simulink model "trocador_PS_GPC_sim"  (R2020a)
settings: Solver=VariableStepAuto  StartTime=0.0  StopTime=tsim  MaxStep=0.01  RelTol=1e-3
values from neighbouring files (symbols this model uses):
  amppert = 0.3    [trocador_PS_GPC.m]
  amppert2 = -0.1    [trocador_PS_GPC.m]
  ampref = 0.5    [trocador_PS_GPC.m]
  F = Ftemp    [trocador_PS_GPC.m]
  H = cell2mat(H)    [trocador_PS_GPC.m]
  Kgpc1 = [Kgpc1; Kgpc(sum(Nu(1:i-1))+1,:)]    [trocador_PS_GPC.m]
  tpert = 15    [trocador_PS_GPC.m]
  tpert2 = 25    [trocador_PS_GPC.m]
  tref = 4    [trocador_PS_GPC.m]
  Ts = 0.15    [trocador_PS_GPC.m]
  zr = blkdiag(zr,ones(N(i),1))    [trocador_PS_GPC.m]
libraries: cstblocks x8
settings Model: Creator=treezao  LastModifiedBy=treezao

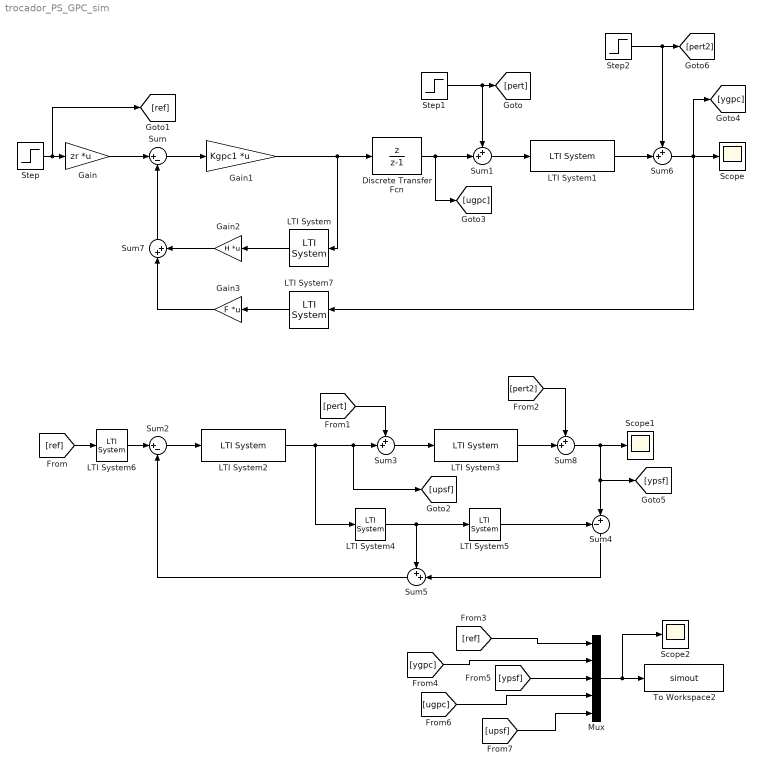
== system trocador_PS_GPC_sim ==
  Discrete Transfer Fcn : DiscreteTransferFcn  Numerator=[1 0]  Denominator=[1 -1]  SampleTime=Ts
  Gain : Gain  Gain=zr  Multiplication=Matrix(K*u)
  Gain1 : Gain  Gain=Kgpc1  Multiplication=Matrix(K*u)
  Gain2 : Gain  Gain=H  Multiplication=Matrix(K*u)
  Gain3 : Gain  Gain=F  Multiplication=Matrix(K*u)
  LTI System : cstblocks/LTI System  sys=zu  IC=[]
  LTI System1 : cstblocks/LTI System  sys=P  IC=[]
  LTI System2 : cstblocks/LTI System  sys=Czps  IC=[]
  LTI System3 : cstblocks/LTI System  sys=P  IC=[]
  LTI System4 : cstblocks/LTI System  sys=Gnz  IC=[]
  LTI System5 : cstblocks/LTI System  sys=Lnz  IC=[]
  LTI System6 : cstblocks/LTI System  sys=Fzps  IC=[]
  LTI System7 : cstblocks/LTI System  sys=zy  IC=[]
  Mux : Mux  Inputs=5
  Scope : Scope
  Scope1 : Scope
  Scope2 : Scope
  Step : Step  Time=tref  After=ampref  SampleTime=0
  Step1 : Step  Time=tpert  After=amppert  SampleTime=0
  Step2 : Step  Time=tpert2  After=amppert2  SampleTime=0
  Sum : Sum  Inputs=|+-
  Sum{1,3,5..6,8} (5 alike) : Sum  Inputs=++|
  Sum2 : Sum  Inputs=|+-
  Sum4 : Sum  Inputs=-+|
  Sum7 : Sum  Inputs=|++
  To Workspace2 : ToWorkspace  VariableName=simout  SampleTime=-1
  wires:
  Step/1 -> [ref], Gain/1
  Sum/1 -> Gain1/1
  Gain1/1 -> LTI System/1, Discrete Transfer Fcn/1
  Step1/1 -> Sum1/1, [pert]
  Sum1/1 -> LTI System1/1
  Sum2/1 -> LTI System2/1
  [ref] -> LTI System6/1
  LTI System2/1 -> [upsf], Sum3/2, LTI System4/1
  Sum3/1 -> LTI System3/1
  [pert] -> Sum3/1
  LTI System4/1 -> Sum5/1, LTI System5/1
  LTI System5/1 -> Sum4/1
  Sum4/1 -> Sum5/2
  Sum5/1 -> Sum2/2
  Mux/1 -> Scope2/1, To Workspace2/1
  [ref] -> Mux/1
  [ygpc] -> Mux/2
  [ypsf] -> Mux/3
  [ugpc] -> Mux/4
  [upsf] -> Mux/5
  Step2/1 -> Sum6/1, [pert2]
  LTI System1/1 -> Sum6/2
  Sum6/1 -> LTI System7/1, [ygpc], Scope/1
  LTI System6/1 -> Sum2/1
  Gain/1 -> Sum/1
  Discrete Transfer Fcn/1 -> [ugpc], Sum1/2
  Sum7/1 -> Sum/2
  Gain2/1 -> Sum7/2
  LTI System/1 -> Gain2/1
  Gain3/1 -> Sum7/1
  LTI System7/1 -> Gain3/1
  LTI System3/1 -> Sum8/2
  Sum8/1 -> Sum4/2, [ypsf], Scope1/1
  [pert2] -> Sum8/1
